simulink model "modelsim"  (R2022a)
settings: Solver=ode1  StartTime=0.0  StopTime=TF  FixedStep=0.0333  RelTol=1e-3
values from neighbouring files (symbols this model uses):
  Hc = 500    [Gierdaempfer.m]    (also in compareData.m; gierUE.m; hoehenregler.m; rolllage.m)
  initpos = [0;0;500]    [init_model.m]
  k_eta_q = 5    [Gierdaempfer.m]    (also in compareData.m; gierUE.m; hoehenregler.m = 10; nickdaempfer.m = 12)
  k_eta_theta = 20    [Gierdaempfer.m]    (also in compareData.m; gierUE.m; hoehenregler.m = 5; nickdaempfer.m = 5)
  k_f_V = 0.01    [Gierdaempfer.m]    (also in compareData.m; gierUE.m; rolllage.m)
  k_theta_H = 0.009    [Gierdaempfer.m]    (also in compareData.m; gierUE.m; hoehenregler.m = 0; rolllage.m)
  k_xi_p = 0.3    [compareData.m]    (also in rolllage.m)
  k_xi_phi = -1.    (= -1)    [compareData.m]    (also in rolllage.m)
  k_zeta_beta = -20    [compareData.m]    (also in rolllage.m)
  k_zeta_r = 30    [Gierdaempfer.m]    (also in compareData.m; rolllage.m)
  phi_c = 10*pi/180    (= 0.174532925199)    [compareData.m]    (also in rolllage.m)
  r_f_V = 0.1    [Gierdaempfer.m]    (also in compareData.m; gierUE.m; rolllage.m)
  T = 0.1/i    [Gierdaempfer.m]    (also in compareData.m = 0.1; rolllage.m = 0.1)
  Vc = 100    [Gierdaempfer.m]    (also in compareData.m; gierUE.m; rolllage.m)
  x0 = [ 85 ... (first row only)    [init_model.m]
libraries: slpidlib x1
settings Model: Creator=Kevin  LastModifiedBy=Kevin
settings OptimizationCC: OptimizeBlockIOStorage=off  ZeroExternalMemoryAtStartup=off  ZeroInternalMemoryAtStartup=off  OptimizeDataStoreBuffers=off  BusAssignmentInplaceUpdate=off
settings DebuggingCC: SFUnexpectedBacktrackingDiag=warning  SFNoUnconditionalDefaultTransitionDiag=warning
settings RTWCC: GenCodeOnly=on  GenerateReport=on  BuildConfiguration=Debug  LaunchReport=on  TargetLang=C++
settings CodeAppCC: ForceParamTrailComments=on  MATLABSourceComments=on  EnableCustomComments=on
settings GRTTargetCC: TargetLangStandard=C++11 (ISO)  CombineSignalStateStructs=on  CodeInterfacePackaging=C++ class  SupportVariableSizeSignals=on  MultiInstanceErrorCode=Warning

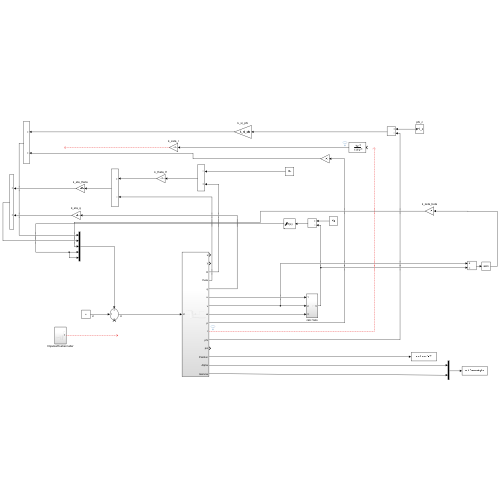
[thumbnail: Simulink's stored preview of the top-level diagram]
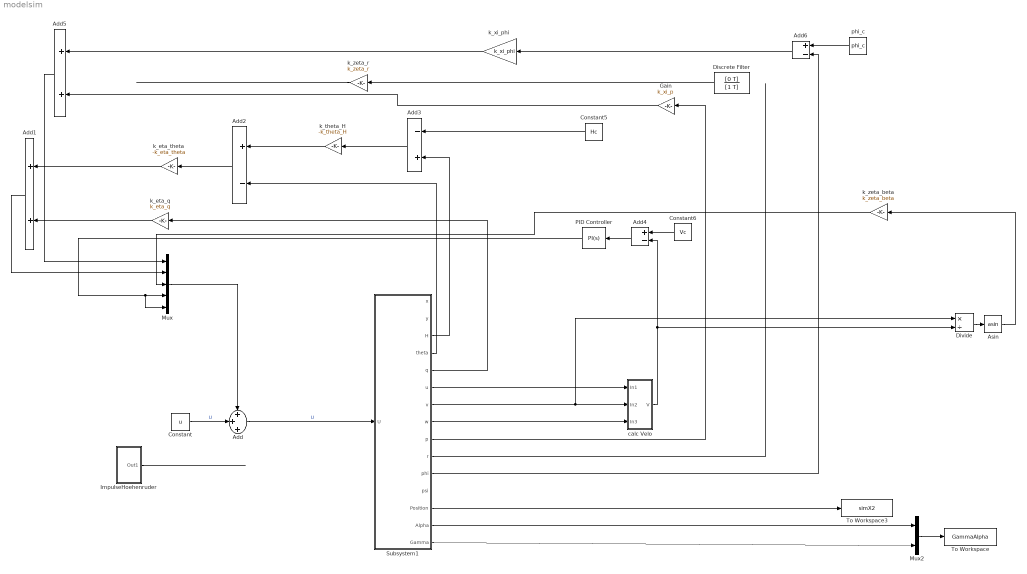
== system modelsim ==
  Add : Sum  Inputs=+++
  Add1 : Sum
  Add2 : Sum  Inputs=+-
  Add3 : Sum  Inputs=-+
  Add4 : Sum  Inputs=+-
  Add5 : Sum
  Add6 : Sum  Inputs=+-
  Asin : Trigonometry  Operator=asin
  Constant : Constant  Value=u
  Constant5 : Constant  Value=Hc
  Constant6 : Constant  Value=Vc
  Discrete Filter : DiscreteFilter  Numerator=[0 T]  Denominator=[1 T]
  Divide : Product  Inputs=*/
  Gain : Gain  Gain=k_xi_p
  ImpulseHoehenruder : Subsystem
  Mux : Mux  Inputs=5
  Mux2 : Mux  Inputs=2
  PID Controller : slpidlib/PID Controller  Controller=PI  Form=Parallel  TimeDomain=Continuous-time  UseExternalTs=off  SampleTime=-1  IntegratorMethod=Forward Euler  FilterMethod=Forward Euler  ControllerParametersSource=internal  P=r_f_V  I=k_f_V  UseKiTs=off  D=0  N=100  UseFilter=on  TunerSelectOption=Transfer Function Based (PID Tuner App)  InitialConditionSource=internal  InitialConditionForIntegrator=0  InitialConditionForFilter=0  DifferentiatorICPrevScaledInput=0  ExternalReset=none  TrackingMode=off  Kt=1  LimitOutput=on  SatLimitsSource=internal  UpperSaturationLimit=inf  LowerSaturationLimit=-inf  LinearizeAsGain=on  AntiWindupMode=none  Kb=1  POutMin=[]  POutMax=[]  IOutMin=[]  IOutMax=[]  DOutMin=[]  DOutMax=[]  NOutMin=[]  NOutMax=[]  SumOutMin=[]  SumOutMax=[]  SaturationOutMin=[]  SaturationOutMax=[]  PParamMin=[]  PParamMax=[]  IParamMin=[]  IParamMax=[]  DParamMin=[]  DParamMax=[]  NParamMin=[]  NParamMax=[]  KbParamMin=[]  KbParamMax=[]  KtParamMin=[]  KtParamMax=[]  KbOutMin=[]  KbOutMax=[]  KtOutMin=[]  KtOutMax=[]  IntegratorOutMin=[]  IntegratorOutMax=[]  FilterOutMin=[]  FilterOutMax=[]  SumI1OutMin=[]  SumI1OutMax=[]  SumI2OutMin=[]  SumI2OutMax=[]  SumI3OutMin=[]  SumI3OutMax=[]  SumI4OutMin=[]  SumI4OutMax=[]  SumDOutMin=[]  SumDOutMax=[]  DifferentiatorOutMin=[]  DifferentiatorOutMax=[]  FilterDiffOutCoefMin=[]  FilterDiffOutCoefMax=[]  ReciprocalOutMin=[]  ReciprocalOutMax=[]  SumDenOutMin=[]  SumDenOutMax=[]  SumNumOutMin=[]  SumNumOutMax=[]  DivideOutMin=[]  DivideOutMax=[]  UdiffTsProdOutMin=[]  UdiffTsProdOutMax=[]  NTsProdOutMin=[]  NTsProdOutMax=[]  UintegralTsProdOutMin=[]  UintegralTsProdOutMax=[]  UngainTsProdOutMin=[]  UngainTsProdOutMax=[]  IntegratorContinuousStateAttributes=''  IntegratorStateMustResolveToSignalObject=off  IntegratorRTWStateStorageClass=Auto  FilterContinuousStateAttributes=''  FilterStateMustResolveToSignalObject=off  FilterRTWStateStorageClass=Auto  ParallelPVariant=InternalParameters  IdealPVariant=Disabled  IVariant=InternalParameters  DVariant=Disabled  IntegratorVariant=Continuous  SatVariant=Enabled  AWVariant=Passthrough  PCopyVariant=Disabled  TRVariant=Disabled  FdbkBlocksVariant=Forward  IdealPFdbkVariant=Disabled  SatFdbkVariant=Disabled  DerivativeFilterVariant=Disabled  NVariant=Disabled  NCopyVariant=Disabled_SignalSpec  FilterICVariant=Disabled  IntegratorICVariant=InternalICs  ExternalResetVariant=Disabled  TRSumVariant=Passthrough  SumFdbkVariant=Disabled  SumVariant=Sum_PI  TsampFilterVariant=InternalTs  TsampNgainVariant=Passthrough  TsampIntegralVariant=Passthrough  ExternalSaturationOutDataTypeStr=Inherit: Same as second input  aMode=0
  Subsystem1 : Subsystem
  To Workspace : ToWorkspace  VariableName=GammaAlpha  SaveFormat=Structure With Time  SampleTime=-1
  To Workspace3 : ToWorkspace  VariableName=simX2  SaveFormat=Structure With Time  SampleTime=-1
  calc Velo : Subsystem
  k_eta_q : Gain  Gain=k_eta_q
  k_eta_theta : Gain  Gain=-k_eta_theta
  k_theta_H : Gain  Gain=-k_theta_H
  k_xi_phi : Gain  Gain=k_xi_phi
  k_zeta_beta : Gain  Gain=k_zeta_beta
  k_zeta_r : Gain  Gain=k_zeta_r
  phi_c : Constant  Value=phi_c
  wires:
  Mux2/1 -> To Workspace/1
  Constant5/1 -> Add3/1
  Add3/1 -> k_theta_H/1
  k_eta_theta/1 -> Add1/1
  PID Controller/1 -> Mux/4, Mux/5
  k_zeta_r/1 -> ?
  Add2/1 -> k_eta_theta/1
  k_eta_q/1 -> Add1/2
  Add1/1 -> Mux/2
  Subsystem1/4(theta) -> Add2/2
  Subsystem1/5(q) -> k_eta_q/1
  Subsystem1/3(H) -> Add3/2
  Subsystem1/13(Position) -> To Workspace3/1
  Subsystem1/14(Alpha) -> Mux2/1
  Subsystem1/15(Gamma) -> Mux2/2
  k_theta_H/1 -> Add2/1
  Subsystem1/6(u) -> calc Velo/1(In1)
  Subsystem1/7(v) -> Divide/1, calc Velo/2(In2)
  Subsystem1/8(w) -> calc Velo/3(In3)
  calc Velo/1(V) -> Divide/2, Add4/2
  Constant6/1 -> Add4/1
  Add4/1 -> PID Controller/1
  Constant/1 -> Add/2  "U"
  Add/1 -> Subsystem1/1(U)  "U"
  Mux/1 -> Add/1
  ImpulseHoehenruder/1(Out1) -> ?
  Subsystem1/10(r) -> ?
  Discrete Filter/1 -> k_zeta_r/1
  Subsystem1/9(p) -> Gain/1
  Gain/1 -> Add5/2
  phi_c/1 -> Add6/1
  Add6/1 -> k_xi_phi/1
  k_xi_phi/1 -> Add5/1
  Add5/1 -> Mux/1
  Subsystem1/11(phi) -> Add6/2
  Divide/1 -> Asin/1
  Asin/1 -> k_zeta_beta/1
  k_zeta_beta/1 -> Mux/3

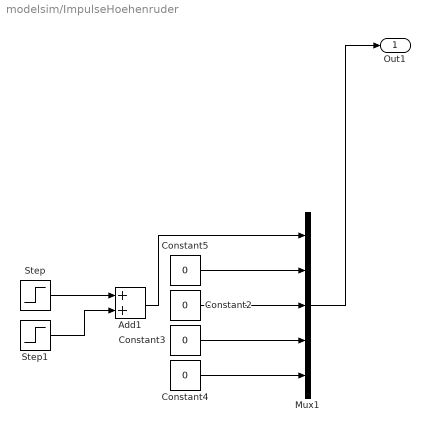
== system modelsim/ImpulseHoehenruder ==
  Add1 : Sum
  Constant{2..5} (4 alike) : Constant  Value=0
  Mux1 : Mux  Inputs=5
  Step : Step  Time=10  After=1*pi/180  SampleTime=0
  Step1 : Step  Time=12  After=-1*pi/180  SampleTime=0
  Out1 : Outport
  wires:
  Step1/1 -> Add1/2
  Mux1/1 -> Out1/1
  Add1/1 -> Mux1/1
  Constant5/1 -> Mux1/2
  Step/1 -> Add1/1
  Constant4/1 -> Mux1/5
  Constant3/1 -> Mux1/4
  Constant2/1 -> Mux1/3

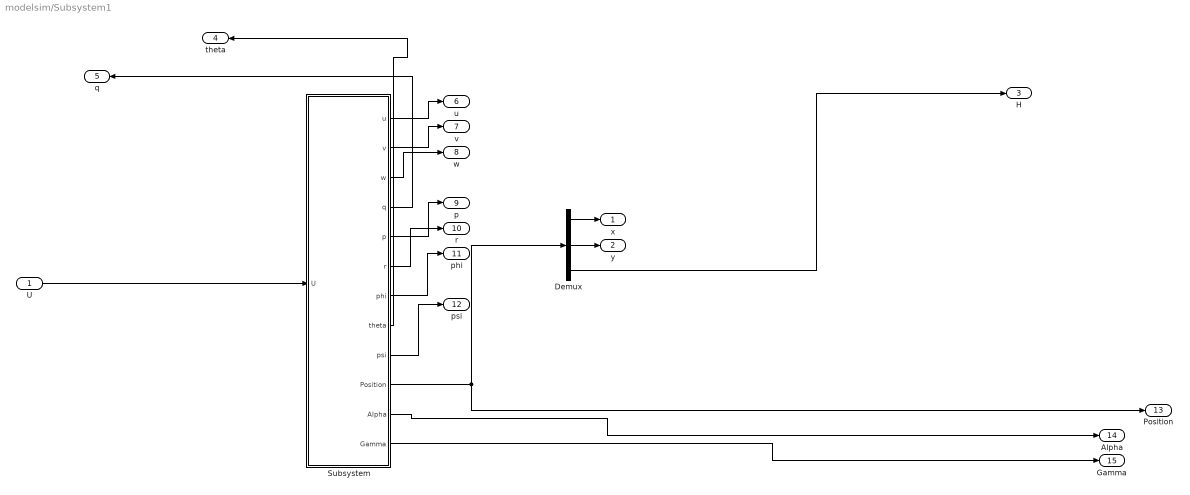
== system modelsim/Subsystem1 ==
  U : Inport
  Demux : Demux  Outputs=3
  Subsystem : Subsystem
  x : Outport
  y : Outport  Port=2
  H : Outport  Port=3
  theta : Outport  Port=4
  q : Outport  Port=5
  u : Outport  Port=6
  v : Outport  Port=7
  w : Outport  Port=8
  p : Outport  Port=9
  r : Outport  Port=10
  phi : Outport  Port=11
  psi : Outport  Port=12
  Position : Outport  Port=13
  Alpha : Outport  Port=14
  Gamma : Outport  Port=15
  wires:
  Subsystem/11(Alpha) -> Alpha/1
  Subsystem/9(psi) -> psi/1
  Subsystem/7(phi) -> phi/1
  Subsystem/10(Position) -> Demux/1, Position/1
  U/1 -> Subsystem/1(U)
  Subsystem/4(q) -> q/1
  Subsystem/8(theta) -> theta/1
  Subsystem/1(u) -> u/1
  Demux/3 -> H/1
  Subsystem/3(w) -> w/1
  Subsystem/5(p) -> p/1
  Subsystem/6(r) -> r/1
  Subsystem/12(Gamma) -> Gamma/1
  Demux/1 -> x/1
  Subsystem/2(v) -> v/1
  Demux/2 -> y/1

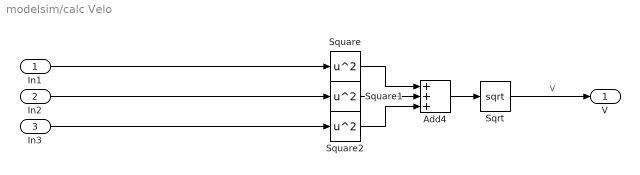
== system modelsim/calc Velo ==
  In1 : Inport
  In2 : Inport  Port=2
  In3 : Inport  Port=3
  Add4 : Sum  Inputs=+++
  Sqrt : Sqrt
  Square : Math  Operator=square
  Square1 : Math  Operator=square
  Square2 : Math  Operator=square
  V : Outport
  wires:
  Square1/1 -> Add4/2
  In3/1 -> Square2/1
  In1/1 -> Square/1
  Square2/1 -> Add4/3
  Add4/1 -> Sqrt/1
  Sqrt/1 -> V/1  "V"
  Square/1 -> Add4/1
  In2/1 -> Square1/1

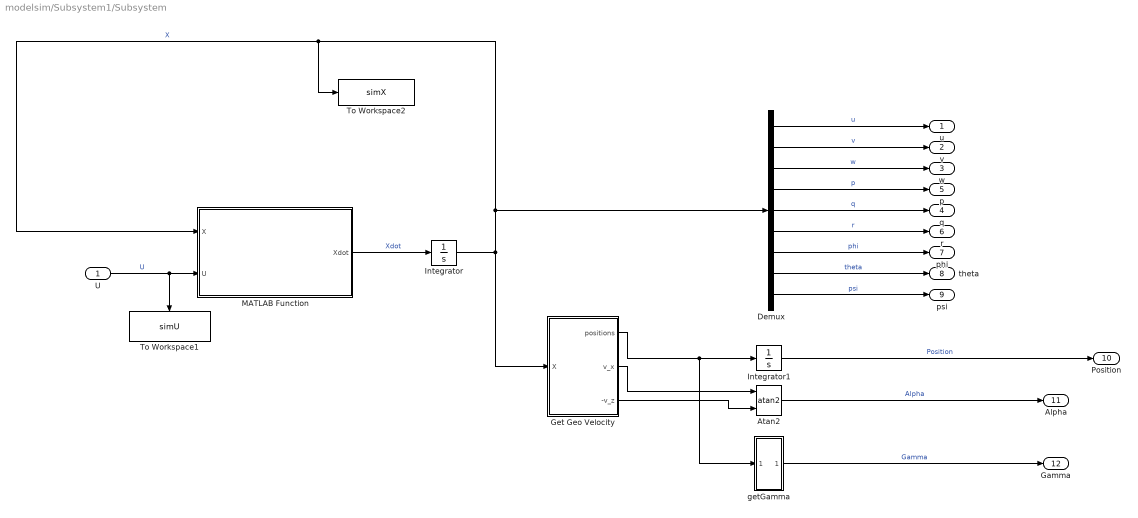
== system modelsim/Subsystem1/Subsystem ==
  U : Inport
  Atan2 : Trigonometry  Operator=atan2
  Demux : Demux  Outputs=9
  Get Geo Velocity : Subsystem
  Integrator : Integrator  InitialCondition=x0
  Integrator1 : Integrator  InitialCondition=initpos
  MATLAB Function : MATLAB Function  TreatAsAtomicUnit=on
  To Workspace1 : ToWorkspace  VariableName=simU  SaveFormat=Structure With Time  SampleTime=-1
  To Workspace2 : ToWorkspace  VariableName=simX  SaveFormat=Structure With Time  SampleTime=-1
  getGamma : Subsystem
  u : Outport
  v : Outport  Port=2
  w : Outport  Port=3
  q : Outport  Port=4
  p : Outport  Port=5
  r : Outport  Port=6
  phi : Outport  Port=7
  theta : Outport  Port=8
  psi : Outport  Port=9
  Position : Outport  Port=10
  Alpha : Outport  Port=11
  Gamma : Outport  Port=12
  wires:
  MATLAB Function/1(Xdot) -> Integrator/1  "Xdot"
  Demux/9 -> psi/1  "psi"
  Demux/7 -> phi/1  "phi"
  Integrator/1 -> To Workspace2/1, MATLAB Function/1(X), Demux/1, Get Geo Velocity/1(X)  "X"
  Demux/8 -> theta/1  "theta"
  Get Geo Velocity/2(v_x) -> Atan2/1
  Get Geo Velocity/1(positions) -> getGamma/1(In1), Integrator1/1
  Get Geo Velocity/3(-v_z) -> Atan2/2
  Demux/2 -> v/1  "v"
  Demux/1 -> u/1  "u"
  Integrator1/1 -> Position/1  "Position"
  Demux/3 -> w/1  "w"
  Atan2/1 -> Alpha/1  "Alpha"
  Demux/6 -> r/1  "r"
  getGamma/1(Out1) -> Gamma/1  "Gamma"
  Demux/4 -> p/1  "p"
  Demux/5 -> q/1  "q"
  U/1 -> MATLAB Function/2(U), To Workspace1/1  "U"

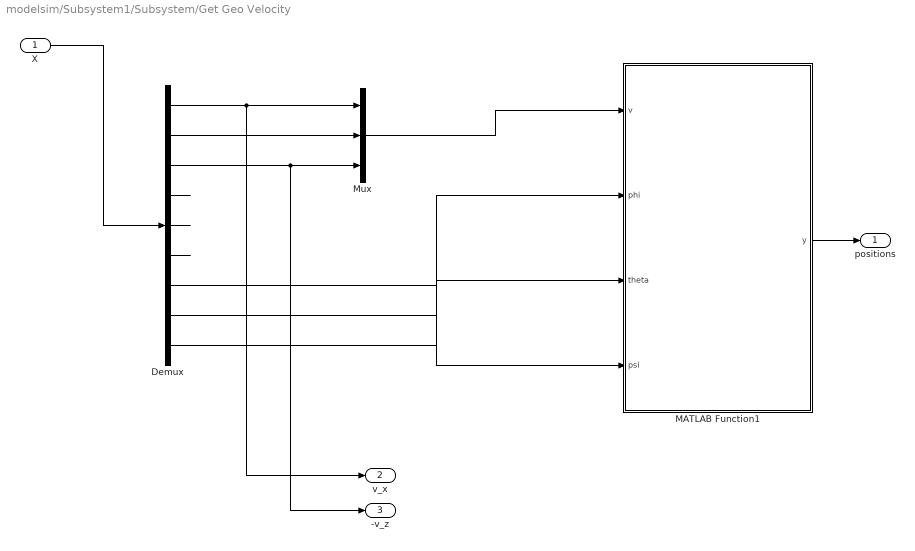
== system modelsim/Subsystem1/Subsystem/Get Geo Velocity ==
  X : Inport
  Demux : Demux  Outputs=9
  MATLAB Function1 : MATLAB Function  TreatAsAtomicUnit=on
  Mux : Mux  Inputs=3
  positions : Outport
  v_x : Outport  Port=2
  -v_z : Outport  Port=3
  wires:
  Demux/9 -> MATLAB Function1/2(phi)
  Demux/4 -> ?
  Mux/1 -> MATLAB Function1/1(v)
  Demux/1 -> v_x/1, Mux/1
  Demux/3 -> -v_z/1, Mux/3
  Demux/5 -> ?
  Demux/7 -> MATLAB Function1/4(psi)
  Demux/8 -> MATLAB Function1/3(theta)
  MATLAB Function1/1(y) -> positions/1
  Demux/2 -> Mux/2
  X/1 -> Demux/1
  Demux/6 -> ?

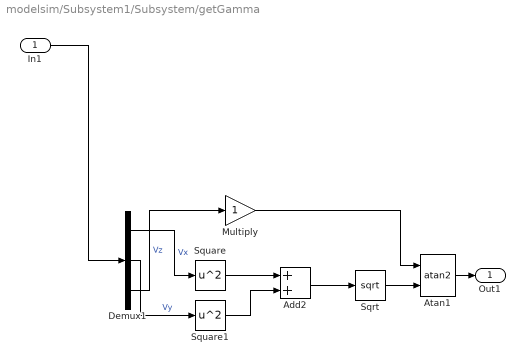
== system modelsim/Subsystem1/Subsystem/getGamma ==
  In1 : Inport
  Add2 : Sum
  Atan1 : Trigonometry  Operator=atan2
  Demux1 : Demux  Outputs=3
  Multiply : Gain
  Sqrt : Sqrt
  Square : Math  Operator=square
  Square1 : Math  Operator=square
  Out1 : Outport
  wires:
  Demux1/2 -> Square1/1  "Vy"
  Sqrt/1 -> Atan1/2
  Multiply/1 -> Atan1/1
  Demux1/1 -> Square/1  "Vx"
  Demux1/3 -> Multiply/1  "Vz"
  Square1/1 -> Add2/2
  Add2/1 -> Sqrt/1
  Square/1 -> Add2/1
  In1/1 -> Demux1/1
  Atan1/1 -> Out1/1

== matlab function modelsim/Subsystem1/Subsystem/Get Geo Velocity/MATLAB Function1 ==
  data: v input; phi input; theta input; y output; psi input
function y  = getpositionwrapper(v,phi,theta,psi)
y = getposition(v,phi,theta,psi);

== matlab function modelsim/Subsystem1/Subsystem/MATLAB Function ==
  data: X input; Xdot output; U input
function Xdot  = aircraft_model_wrapper(X,U)
  Xdot = aircraft_model(X,U);
end
